simulink model "imcn"  (Simulink 6.5)
settings: Solver=ode45  SolverMode=SingleTasking  StartTime=0.0  StopTime=999999  MaxStep=10  RelTol=1e-3  AbsTol=1e-3
settings Model: Creator=lfd  LastModifiedBy=lfd  ExtModeAutoUpdateStatusClock=off
settings DataIOCC: LimitDataPoints=off  SaveOutput=off  SaveTime=off
settings OptimizationCC: BlockReduction=off  BooleanDataType=off
settings DebuggingCC: SolverPrmCheckMsg=none  MultiTaskDSMMsg=warning  MultiTaskCondExecSysMsg=none  StrictBusMsg=None
settings HardwareCC: TargetUnknown=on
settings RTWCC: IncludeERTFirstTime=on
settings GRTTargetCC: ModelReferenceCompliant=off  MatFileLogging=off

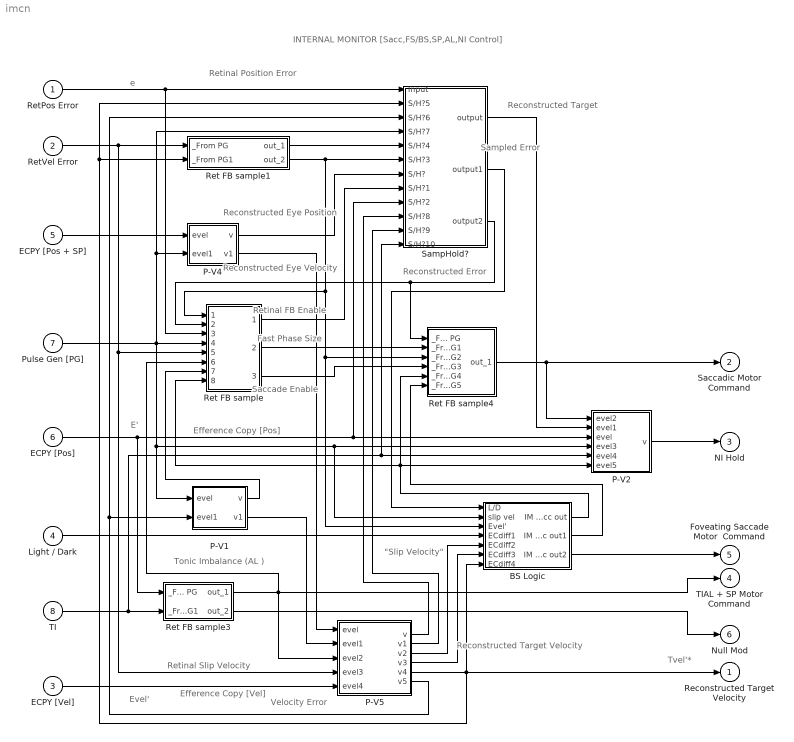
== system imcn ==
  note: E'
  note: Tonic Imbalance (AL )
  note: Reconstructed
      | Target Velocity
  note: Retinal FB
      | Enable
  note: Saccade
      | Enable
  note: Fast Phase
      | Size
  note: Sampled
      | Error
  note: Reconstructed
      | Target
  note: Reconstructed
      | Error
  note: Evel'
  note: Tvel'*
  note: INTERNAL MONITOR [Sacc,FS/BS,SP,AL,NI Control]
  note: Velocity Error
  note: "Slip Velocity"
  note: e
  note: Reconstructed
      | Eye Position
  note: Reconstructed
      | Eye Velocity
  note: Retinal Slip Velocity
  note: Retinal Position Error
  note: Efference Copy [Vel]
  note: Efference Copy [Pos]
  RetPos Error : Inport
  RetVel Error : Inport  Port=2
  ECPY [Vel] : Inport  Port=3
  Light / Dark : Inport  Port=4
  ECPY [Pos + SP] : Inport  Port=5
  ECPY [Pos] : Inport  Port=6
  Pulse Gen [PG] : Inport  Port=7
  TI : Inport  Port=8
  BS Logic : Subsystem
      mask Display: disp('Braking/Foveating\nSaccade\nLogic')
  P-V1 : Subsystem
      mask Display: disp('Saccade\n& Drift\nBlanking')
  P-V2 : Subsystem
      mask Display: disp('NI\nControl')
  P-V4 : Subsystem
      mask Display: disp('Model\nPlant+')
  P-V5 : Subsystem
      mask Display: disp('Target &\nSlip Velocity\nReconstruction')
  Ret FB sample : Subsystem
      mask Display: disp('Saccade\nEnable')
  Ret FB sample1 : Subsystem
      mask Display: disp('Target Change\nDetection')
  Ret FB sample3 : Subsystem
      mask Display: disp('Alexander''s\nLaw')
  Ret FB sample4 : Subsystem
      mask Display: disp('Saaccade\nMotor\nCommand')
  SampHold? : Subsystem
      mask Display: disp('Sampled\nTarget & Error\nReconstruction')
  Reconstructed Target Velocity : Outport  InitialOutput=0
  Saccadic Motor Command : Outport  Port=2  InitialOutput=0
  NI Hold : Outport  Port=3  InitialOutput=0
  TIAL + SP Motor Command : Outport  Port=4  InitialOutput=0
  Foveating Saccade Motor  Command : Outport  Port=5  InitialOutput=0
  Null Mod : Outport  Port=6  InitialOutput=0
  wires:
  RetPos Error/1 -> Ret FB sample/3(_From PG3), SampHold?/1(Input)
  ECPY [Pos + SP]/1 -> P-V4/1(evel)
  P-V4/1(v) -> SampHold?/7(S/H?)
  P-V2/1(v) -> NI Hold/1
  Ret FB sample/2(out_2) -> Ret FB sample4/2(_From PG1)
  Pulse Gen [PG]/1 -> Ret FB sample/4(_From PG1), P-V1/1(evel), P-V2/4(evel3), BS Logic/2(slip vel), P-V4/2(evel1), SampHold?/4(S/H?7)
  Ret FB sample/1(out_1) -> SampHold?/8(S/H?1)
  TI/1 -> Ret FB sample3/2(_From PG1), P-V2/5(evel4), SampHold?/12(S/H?10)
  Ret FB sample3/1(out_1) -> Ret FB sample/6(_From PG4), P-V5/3(evel2), TIAL + SP Motor Command/1
  P-V5/1(v) -> SampHold?/10(S/H?8)
  P-V5/2(v1) -> SampHold?/11(S/H?9)
  BS Logic/3(IM Sacc out2) -> Foveating Saccade Motor  Command/1
  P-V5/4(v3) -> BS Logic/6(ECdiff3)
  P-V5/3(v2) -> BS Logic/5(ECdiff2)
  Light / Dark/1 -> BS Logic/4(ECdiff1)
  BS Logic/2(IM Sacc out1) -> Ret FB sample4/6(_From PG5)
  Ret FB sample1/1(out_1) -> SampHold?/5(S/H?4)
  Ret FB sample1/2(out_2) -> SampHold?/6(S/H?3), Ret FB sample/1(_From PG2), BS Logic/3(Evel'), Ret FB sample4/3(_From PG2)
  SampHold?/2(output1) -> BS Logic/1(L/D)
  SampHold?/3(output2) -> Ret FB sample/2(_From PG), Ret FB sample4/1(_From PG)
  P-V5/5(v4) -> Reconstructed Target Velocity/1, Ret FB sample1/2(_From PG1), SampHold?/2(S/H?5), BS Logic/7(ECdiff4)
  P-V4/2(v1) -> P-V5/1(evel)
  P-V1/2(v1) -> P-V5/2(evel1)
  P-V5/6(v5) -> SampHold?/3(S/H?6), P-V1/2(evel1)
  Ret FB sample/3(out_3) -> Ret FB sample4/4(_From PG3)
  Ret FB sample4/1(out_1) -> Saccadic Motor Command/1, P-V2/1(evel2)
  SampHold?/1(output) -> P-V2/2(evel1)
  ECPY [Pos]/1 -> Ret FB sample3/1(_From PG), P-V2/3(evel), SampHold?/9(S/H?2)
  BS Logic/1(IM Sacc out) -> P-V2/6(evel5), Ret FB sample4/5(_From PG4), Ret FB sample/8(_From PG6)
  P-V1/1(v) -> Ret FB sample/7(_From PG7)
  ECPY [Vel]/1 -> P-V5/5(evel4)
  RetVel Error/1 -> Ret FB sample/5(_From PG5), P-V5/4(evel3), Ret FB sample1/1(_From PG)
  Ret FB sample3/2(out_2) -> Null Mod/1

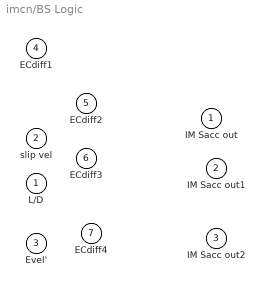
== system imcn/BS Logic ==
  L/D : Inport
  slip vel : Inport  Port=2
  Evel' : Inport  Port=3
  ECdiff1 : Inport  Port=4
  ECdiff2 : Inport  Port=5
  ECdiff3 : Inport  Port=6
  ECdiff4 : Inport  Port=7
  IM Sacc out : Outport  InitialOutput=0
  IM Sacc out1 : Outport  Port=2  InitialOutput=0
  IM Sacc out2 : Outport  Port=3  InitialOutput=0

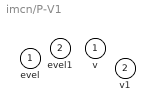
== system imcn/P-V1 ==
  evel : Inport
  evel1 : Inport  Port=2
  v : Outport  InitialOutput=0
  v1 : Outport  Port=2  InitialOutput=0

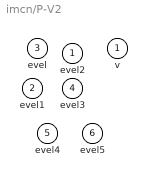
== system imcn/P-V2 ==
  evel2 : Inport
  evel1 : Inport  Port=2
  evel : Inport  Port=3
  evel3 : Inport  Port=4
  evel4 : Inport  Port=5
  evel5 : Inport  Port=6
  v : Outport  InitialOutput=0

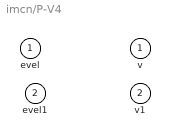
== system imcn/P-V4 ==
  evel : Inport
  evel1 : Inport  Port=2
  v : Outport  InitialOutput=0
  v1 : Outport  Port=2  InitialOutput=0

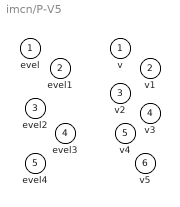
== system imcn/P-V5 ==
  evel : Inport
  evel1 : Inport  Port=2
  evel2 : Inport  Port=3
  evel3 : Inport  Port=4
  evel4 : Inport  Port=5
  v : Outport  InitialOutput=0
  v1 : Outport  Port=2  InitialOutput=0
  v2 : Outport  Port=3  InitialOutput=0
  v3 : Outport  Port=4  InitialOutput=0
  v4 : Outport  Port=5  InitialOutput=0
  v5 : Outport  Port=6  InitialOutput=0

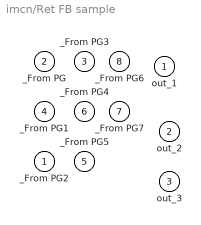
== system imcn/Ret FB sample ==
  _From PG2 : Inport
  _From PG : Inport  Port=2
  _From PG3 : Inport  Port=3
  _From PG1 : Inport  Port=4
  _From PG5 : Inport  Port=5
  _From PG4 : Inport  Port=6
  _From PG7 : Inport  Port=7
  _From PG6 : Inport  Port=8
  out_1 : Outport  InitialOutput=0
  out_2 : Outport  Port=2  InitialOutput=0
  out_3 : Outport  Port=3  InitialOutput=0

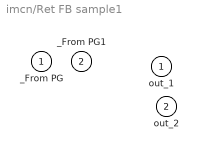
== system imcn/Ret FB sample1 ==
  _From PG : Inport
  _From PG1 : Inport  Port=2
  out_1 : Outport  InitialOutput=0
  out_2 : Outport  Port=2  InitialOutput=0

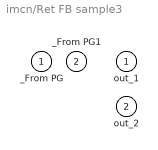
== system imcn/Ret FB sample3 ==
  _From PG : Inport
  _From PG1 : Inport  Port=2
  out_1 : Outport  InitialOutput=0
  out_2 : Outport  Port=2  InitialOutput=0

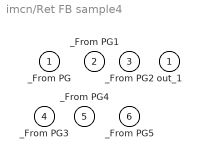
== system imcn/Ret FB sample4 ==
  _From PG : Inport
  _From PG1 : Inport  Port=2
  _From PG2 : Inport  Port=3
  _From PG3 : Inport  Port=4
  _From PG4 : Inport  Port=5
  _From PG5 : Inport  Port=6
  out_1 : Outport  InitialOutput=0

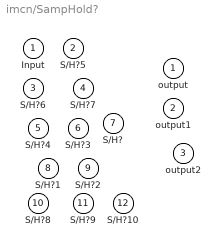
== system imcn/SampHold? ==
  Input : Inport
  S/H?5 : Inport  Port=2
  S/H?6 : Inport  Port=3
  S/H?7 : Inport  Port=4
  S/H?4 : Inport  Port=5
  S/H?3 : Inport  Port=6
  S/H? : Inport  Port=7
  S/H?1 : Inport  Port=8
  S/H?2 : Inport  Port=9
  S/H?8 : Inport  Port=10
  S/H?9 : Inport  Port=11
  S/H?10 : Inport  Port=12
  output : Outport  InitialOutput=0
  output1 : Outport  Port=2  InitialOutput=0
  output2 : Outport  Port=3  InitialOutput=0
